simulink model "estimatetransform"  (R2019b)
settings: Solver=VariableStepAuto  StartTime=0.0  StopTime=10.0  RelTol=1e-3
undefined symbols (not defined in the file or in its folder): matchedPtsDistorted, matchedPtsOriginal
libraries: visiongeotforms x2
settings Model: Creator=zacefron  LastModifiedBy=zacefron

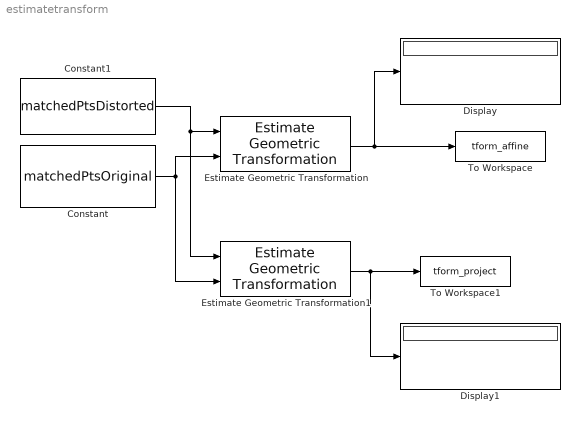
== system estimatetransform ==
  Constant : Constant  Value=matchedPtsOriginal
  Constant1 : Constant  Value=matchedPtsDistorted
  Display : Display
      settings: Decimation=3
  Display1 : Display
      settings: Decimation=3
  Estimate Geometric Transformation : visiongeotforms/Estimate Geometric Transformation  tformType=Affine  isRandomSampling=off  algMethod=Least Median of Squares  distanceAlg=2.5  distanceGeo=2.5  numMethod=Specified value  sampleNum=500  desiredConfidence=99  maxSampleNum=1000  isStopSampling=off  percentStop=75  isRefineTForm=on  isReleaseMode=on  isOutputInlier=off  outDT4IntInput=Obsolete10a  outDT4IntInputActive=Double  isVarSizeAllowed=on
      settings: SourceProductName=Computer Vision Toolbox  SourceProductBaseCode=VP
  Estimate Geometric Transformation1 : visiongeotforms/Estimate Geometric Transformation  tformType=Projective  isRandomSampling=off  algMethod=Least Median of Squares  distanceAlg=2.5  distanceGeo=2.5  numMethod=Specified value  sampleNum=500  desiredConfidence=99  maxSampleNum=1000  isStopSampling=off  percentStop=75  isRefineTForm=on  isReleaseMode=on  isOutputInlier=off  outDT4IntInput=Obsolete10a  outDT4IntInputActive=Double  isVarSizeAllowed=on
      settings: SourceProductName=Computer Vision Toolbox  SourceProductBaseCode=VP
  To Workspace : ToWorkspace  VariableName=tform_affine  SampleTime=-1
      settings: Save2DSignal=2-D array (concatenate along first dimension)
  To Workspace1 : ToWorkspace  VariableName=tform_project  SampleTime=-1
      settings: Save2DSignal=2-D array (concatenate along first dimension)
  wires:
  Estimate Geometric Transformation/1 -> To Workspace/1, Display/1
  Constant1/1 -> Estimate Geometric Transformation1/1, Estimate Geometric Transformation/1
  Constant/1 -> Estimate Geometric Transformation1/2, Estimate Geometric Transformation/2
  Estimate Geometric Transformation1/1 -> Display1/1, To Workspace1/1
